simulink model "heaveCompMichael_v07"  (R2022b)
settings: Solver=VariableStepAuto  StartTime=0.0  StopTime=20  RelTol=1e-3
model workspace (MATLAB code in the model file):
  | %fluid data
  | rho = 875;
  | %valve config
  | P_r = 70e5;
  | Cd = 0.7;
  | Q_r = 200/6e4;
  | AdMax = Q_r/Cd/sqrt(2/rho*P_r/2);
  | 
  | g = 9.81;                   %gravity
  | zw = 0.8;                   %wave amplitude
  | tw = 10;                    %total wave period
  | ig = 46;                    %gear ratio gearbox
  | m = 9000;                   %mass of payload
  | mueq = 0.15;                %friction coeffisient
  | dd = 0.45;                  %diameter drum
  | nyv = 0.92;                 %volumetric effissiency
  | rd = dd/2;                  %radius drum
  | omega0 = 5;                 %velosity in friction equation
  | omegap = 1500;              %velosity hpu pump
  | nsh = 3;
  | gearrationsh = nsh.*2;
libraries: fl_lib x30, nesl_utility x18, sh_lib x4, slpidlib x1
settings Model: Creator=tolla  LastModifiedBy=marcu
settings SolverCC: MaxConsecutiveMinStep=10
settings DebuggingCC: UnconnectedInputMsg=warning  UnconnectedOutputMsg=warning  UnconnectedLineMsg=warning
settings ModelReferenceCC: EnableRefExpFcnMdlSchedulingChecks=on
settings RTWCC: DLArmComputeVersion=19.05

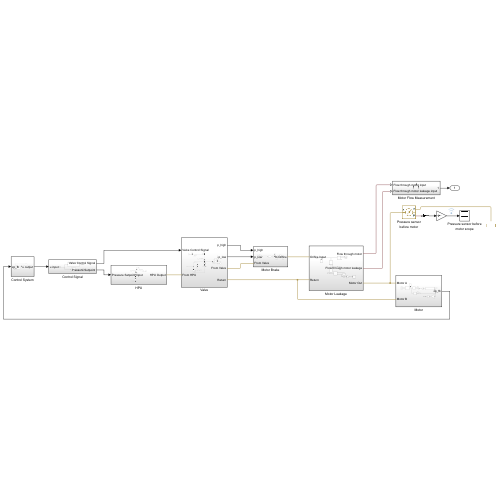
[thumbnail: Simulink's stored preview of the top-level diagram]
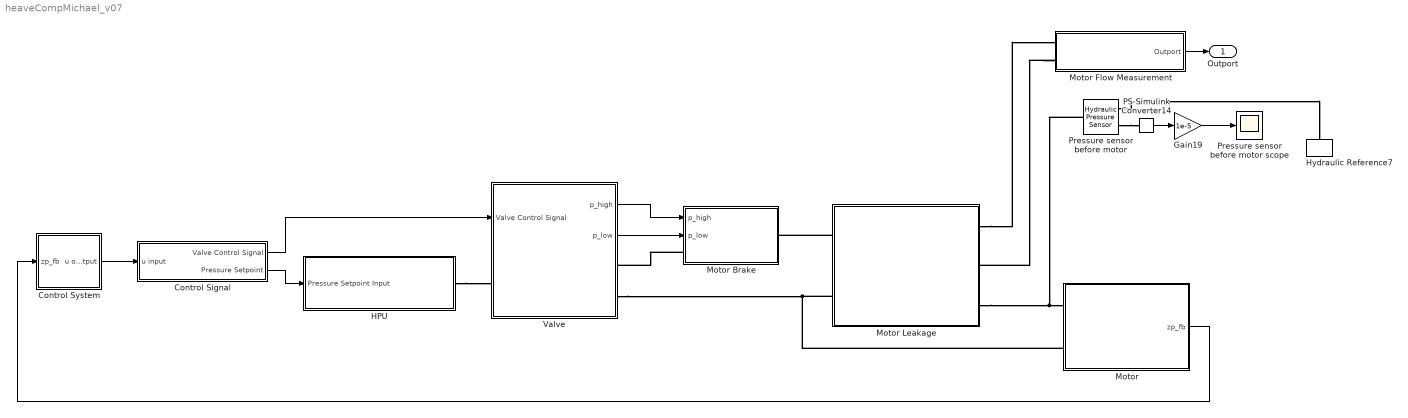
== system heaveCompMichael_v07 ==
  Control Signal : Subsystem
  Control System : Subsystem
  Gain19 : Gain  Gain=1e-5
  HPU : Subsystem
  Hydraulic Reference7 : fl_lib/Hydraulic/Hydraulic Elements/Hydraulic Reference
  Motor : Subsystem
  Motor Brake : Subsystem
  Motor Flow Measurement : Subsystem
  Motor Leakage : Subsystem
  PS-Simulink Converter14 : nesl_utility/PS-Simulink Converter  PhysicalDomain=network_engine_domain  SubClassName=ps_output  LeftPortType=input  RightPortType=output  PseudoPeriodic=off  Frequencies=[]  VectorFormat=inherit  Unit=inherit  AffineConversion=off
  Pressure sensor before motor : fl_lib/Hydraulic/Hydraulic Sensors/Hydraulic Pressure Sensor
  Pressure sensor before motor scope : Scope
  Valve : Subsystem
  Outport : Outport
  wires:
  PS-Simulink Converter14/1 -> Gain19/1
  Gain19/1 -> Pressure sensor before motor scope/1
  Motor/1(zp_fb) -> Control System/1(zp_fb)
  Valve/1(p_high) -> Motor Brake/1(p_high)
  Valve/2(p_low) -> Motor Brake/2(p_low)
  Motor Flow Measurement/1(Outport) -> Outport/1
  Control System/1(u output) -> Control Signal/1(u input)
  Control Signal/1(Valve Control Signal) -> Valve/1(Valve Control Signal)
  Control Signal/2(Pressure Setpoint) -> HPU/1(Pressure Setpoint Input)
  connections:
  Pressure sensor before motor/RConn1 -- Hydraulic Reference7/LConn1
  Pressure sensor before motor/RConn2 -- PS-Simulink Converter14/LConn1
  Motor/LConn2 -- Valve/RConn2 -- Motor Leakage/LConn2
  Motor Brake/LConn1 -- Valve/RConn1
  HPU/RConn1 -- Valve/LConn1
  Pressure sensor before motor/LConn1 -- Motor Leakage/RConn3 -- Motor/LConn1
  Motor Leakage/LConn1 -- Motor Brake/RConn1
  Motor Leakage/RConn1 -- Motor Flow Measurement/LConn1
  Motor Flow Measurement/LConn2 -- Motor Leakage/RConn2

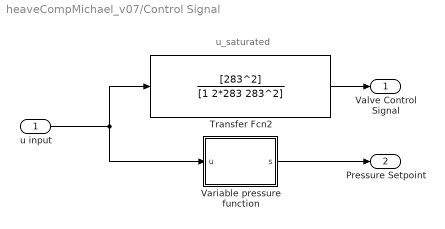
== system heaveCompMichael_v07/Control Signal ==
  note: u_saturated
  u input : Inport
  Transfer Fcn2 : TransferFcn  Numerator=[283^2]  Denominator=[1 2*283 283^2]
  Variable pressure function : MATLAB Function  TreatAsAtomicUnit=on
  Valve Control Signal : Outport
  Pressure Setpoint : Outport  Port=2
  wires:
  u input/1 -> Variable pressure function/1(u), Transfer Fcn2/1
  Variable pressure function/1(s) -> Pressure Setpoint/1
  Transfer Fcn2/1 -> Valve Control Signal/1

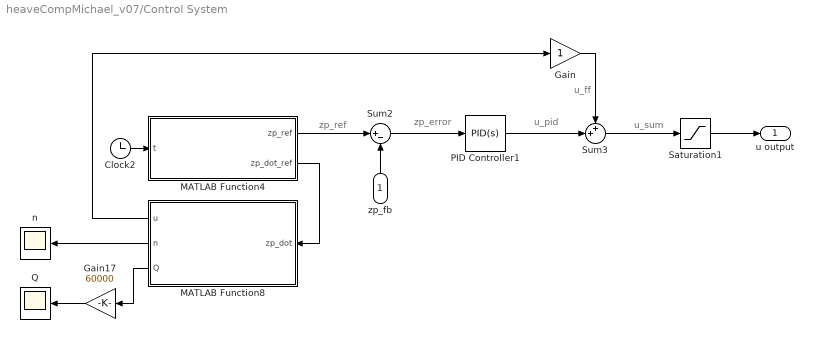
== system heaveCompMichael_v07/Control System ==
  note: u_ff
  note: u_sum
  note: u_pid
  note: zp_error
  note: zp_ref
  zp_fb : Inport
  Clock2 : Clock
  Gain : Gain
  Gain17 : Gain  Gain=60000
  MATLAB Function4 : MATLAB Function  TreatAsAtomicUnit=on
  MATLAB Function8 : MATLAB Function  TreatAsAtomicUnit=on
  PID Controller1 : slpidlib/PID Controller  Controller=PID  Form=Parallel  TimeDomain=Continuous-time  UseExternalTs=off  SampleTime=-1  IntegratorMethod=Forward Euler  FilterMethod=Forward Euler  ControllerParametersSource=internal  P=20  I=0  UseKiTs=off  D=0  N=100  UseFilter=on  TunerSelectOption=Transfer Function Based (PID Tuner App)  InitialConditionSource=internal  InitialConditionForIntegrator=0  InitialConditionForFilter=0  DifferentiatorICPrevScaledInput=0  ExternalReset=none  TrackingMode=off  Kt=1  LimitOutput=off  SatLimitsSource=internal  UpperSaturationLimit=inf  LowerSaturationLimit=-inf  LinearizeAsGain=on  AntiWindupMode=none  Kb=1  LimitIntegrator=off  UpperIntegratorSaturationLimit=inf  LowerIntegratorSaturationLimit=-inf  POutMin=[]  POutMax=[]  IOutMin=[]  IOutMax=[]  DOutMin=[]  DOutMax=[]  NOutMin=[]  NOutMax=[]  SumOutMin=[]  SumOutMax=[]  SaturationOutMin=[]  SaturationOutMax=[]  PParamMin=[]  PParamMax=[]  IParamMin=[]  IParamMax=[]  DParamMin=[]  DParamMax=[]  NParamMin=[]  NParamMax=[]  KbParamMin=[]  KbParamMax=[]  KtParamMin=[]  KtParamMax=[]  KbOutMin=[]  KbOutMax=[]  KtOutMin=[]  KtOutMax=[]  IntegratorOutMin=[]  IntegratorOutMax=[]  FilterOutMin=[]  FilterOutMax=[]  SumI1OutMin=[]  SumI1OutMax=[]  SumI2OutMin=[]  SumI2OutMax=[]  SumI3OutMin=[]  SumI3OutMax=[]  SumI4OutMin=[]  SumI4OutMax=[]  SumDOutMin=[]  SumDOutMax=[]  DifferentiatorOutMin=[]  DifferentiatorOutMax=[]  FilterDiffOutCoefMin=[]  FilterDiffOutCoefMax=[]  ReciprocalOutMin=[]  ReciprocalOutMax=[]  SumDenOutMin=[]  SumDenOutMax=[]  SumNumOutMin=[]  SumNumOutMax=[]  DivideOutMin=[]  DivideOutMax=[]  UdiffTsProdOutMin=[]  UdiffTsProdOutMax=[]  NTsProdOutMin=[]  NTsProdOutMax=[]  UintegralTsProdOutMin=[]  UintegralTsProdOutMax=[]  UngainTsProdOutMin=[]  UngainTsProdOutMax=[]  ClampingZeroOutDataTypeStr=Inherit: Inherit via back propagation  ClampingZeroOutMin=[]  ClampingZeroOutMax=[]  FilterDenConstantOutDataTypeStr=Inherit: Inherit via back propagation  FilterDenConstantOutMin=[]  FilterDenConstantOutMax=[]  PCopyOutDataTypeStr=Inherit: Inherit via back propagation  PCopyOutMin=[]  PCopyOutMax=[]  NCopyOutDataTypeStr=Inherit: Inherit via back propagation  NCopyOutMin=[]  NCopyOutMax=[]  IntegratorContinuousStateAttributes=''  IntegratorStateMustResolveToSignalObject=off  IntegratorRTWStateStorageClass=Auto  FilterContinuousStateAttributes=''  FilterStateMustResolveToSignalObject=off  FilterRTWStateStorageClass=Auto  ParallelPVariant=InternalParameters  IdealPVariant=Disabled  IVariant=InternalParameters  DVariant=InternalParameters  IntegratorVariant=Continuous  SatVariant=Disabled  AWVariant=Passthrough  PCopyVariant=Disabled  TRVariant=Disabled  FdbkBlocksVariant=Forward  IdealPFdbkVariant=Disabled  SatFdbkVariant=Disabled  DerivativeFilterVariant=ContFilter  NVariant=InternalParameters  NCopyVariant=Disabled  FilterICVariant=InternalICsFilter  IntegratorICVariant=InternalICs  ExternalResetVariant=Disabled  TRSumVariant=Passthrough  SumFdbkVariant=Disabled  SumVariant=Sum_PID  TsampFilterVariant=InternalTs  TsampNgainVariant=Passthrough  TsampIntegralVariant=Passthrough  ExternalSaturationOutDataTypeStr=Inherit: Same as second input
  Q : Scope
  Saturation1 : Saturate  UpperLimit=1  LowerLimit=-1
  Sum2 : Sum  Inputs=|+-
  Sum3 : Sum  Inputs=++|
  n : Scope
  u output : Outport
  wires:
  MATLAB Function8/3(Q) -> Gain17/1
  PID Controller1/1 -> Sum3/2
  MATLAB Function4/2(zp_dot_ref) -> MATLAB Function8/1(zp_dot)
  Gain17/1 -> Q/1
  Clock2/1 -> MATLAB Function4/1(t)
  MATLAB Function8/2(n) -> n/1
  Sum3/1 -> Saturation1/1
  zp_fb/1 -> Sum2/2
  MATLAB Function4/1(zp_ref) -> Sum2/1
  Sum2/1 -> PID Controller1/1
  MATLAB Function8/1(u) -> Gain/1
  Saturation1/1 -> u output/1
  Gain/1 -> Sum3/1

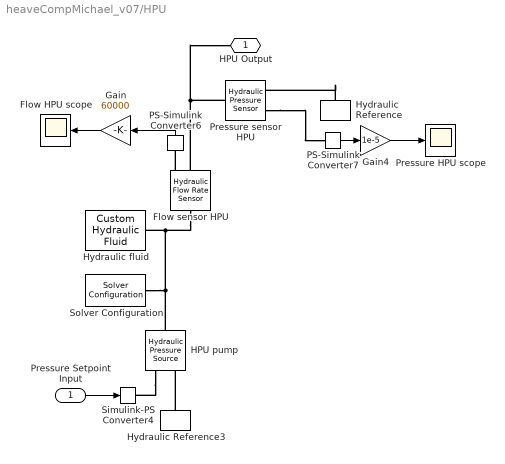
== system heaveCompMichael_v07/HPU ==
  Pressure Setpoint Input : Inport
  Flow HPU scope : Scope
  Flow sensor HPU : fl_lib/Hydraulic/Hydraulic Sensors/Hydraulic Flow Rate Sensor
  Gain : Gain  Gain=60000
  Gain4 : Gain  Gain=1e-5
  HPU pump : fl_lib/Hydraulic/Hydraulic Sources/Hydraulic Pressure Source
      settings: InternalSimscapePortConfiguration="{\"Bottom\":[],\"Left\":[{\"id\":\"P\",\"label\":\"P\",\"type\":\"foundation.hydraulic.hydraulic\"}],\"Right\":[{\"id\":\"S\",\"label\":\"S\",\"type\":\"input\"},{\"id\":\"T\",\"label\":\"T\",\"type\":\"foundation.hydraulic.hydraulic\"}],\"Top\":[]}"
  Hydraulic Reference : fl_lib/Hydraulic/Hydraulic Elements/Hydraulic Reference
  Hydraulic Reference3 : fl_lib/Hydraulic/Hydraulic Elements/Hydraulic Reference
  Hydraulic fluid : fl_lib/Hydraulic/Hydraulic Utilities/Custom Hydraulic Fluid  density=875 kg/m^3  viscosity_kin=18e-6 m^2/s  bulk=1100 MPa  alpha=0.005  range_error=2
      settings: InternalSimscapePortConfiguration="{\"Bottom\":[],\"Left\":[],\"Right\":[{\"id\":\"G\",\"label\":\"\",\"type\":\"foundation.hydraulic.hydraulic\"}],\"Top\":[]}"
  PS-Simulink Converter6 : nesl_utility/PS-Simulink Converter  PhysicalDomain=network_engine_domain  SubClassName=ps_output  LeftPortType=input  RightPortType=output  PseudoPeriodic=off  Frequencies=[]  VectorFormat=inherit  Unit=inherit  AffineConversion=off
  PS-Simulink Converter7 : nesl_utility/PS-Simulink Converter  PhysicalDomain=network_engine_domain  SubClassName=ps_output  LeftPortType=input  RightPortType=output  PseudoPeriodic=off  Frequencies=[]  VectorFormat=inherit  Unit=inherit  AffineConversion=off
  Pressure HPU scope : Scope
  Pressure sensor HPU : fl_lib/Hydraulic/Hydraulic Sensors/Hydraulic Pressure Sensor
  Simulink-PS Converter4 : nesl_utility/Simulink-PS Converter  PhysicalDomain=network_engine_domain  SubClassName=ps_input  LeftPortType=input  RightPortType=output  PseudoPeriodic=off  Frequencies=[]  NoiseDistribution=none  NoiseParameters=[]  Unit=1  AffineConversion=off  FilteringAndDerivatives=provide  SimscapeFilterOrder=1  InputFilterTimeConstant=0.001  UdotUserProvided=0
  Solver Configuration : nesl_utility/Solver Configuration  PhysicalDomain=network_engine_domain  SubClassName=solver  LeftPortType=input  RightPortType=generic  Tones=[]  Harmonics=[]  SimulateNoise=off  Profile=off  UseLocalSampling=off  EnableSwitchedLinearOptims=on  FrequencyDomain=off  UseCCode=off  RelTol=0.001  AbsTol=1e-06  MinStep=1e-09  ToWorkspace=off  RevertToSquareIcSolve=off  NumHomotopyIterations=100  PhasorMode=off  PhasorModeNumHarmonics=1  ConsistencySolver=NEWTON_FTOL  IndexReductionMethod=DerivativeReplacement  DoDC=off  ResidualTolerance=1e-09  ConsistencyTolSource=GLOBAL  ConsistencyAbsTol=0.001  ConsistencyRelTol=0.001  ConsistencyTolFactor=0.001  UseLocalSolver=off  LocalSolverChoice=NE_BACKWARD_EULER_ADVANCER  ResolveIndetEquations=on  FunctionEvalNumThread=1  LocalSolverSampleTime=0.001  DoFixedCost=off  MaxNonlinIter=3  MaxModeIter=2  ComputeImpulses=off  ImpulseIterations=2  LinearAlgebra=auto  LinearAlgebraNumThread=0  EquationFormulation=NE_TIME_EF  DelaysMemoryBudget=1024  AutomaticFiltering=on  FilteringTimeConstant=0.001  PartitionStorageMethod=AS_NEEDED  PartitionMemoryBudget=1024  PartitionMethod=ROBUST
  HPU Output : PMIOPort  Side=Right
  wires:
  PS-Simulink Converter6/1 -> Gain/1
  PS-Simulink Converter7/1 -> Gain4/1
  Pressure Setpoint Input/1 -> Simulink-PS Converter4/1
  Gain/1 -> Flow HPU scope/1
  Gain4/1 -> Pressure HPU scope/1
  connections:
  HPU pump/LConn1 -- Solver Configuration/RConn1 -- Hydraulic fluid/RConn1 -- Flow sensor HPU/LConn1
  Hydraulic Reference3/LConn1 -- HPU pump/RConn2
  HPU pump/RConn1 -- Simulink-PS Converter4/RConn1
  Pressure sensor HPU/RConn2 -- PS-Simulink Converter7/LConn1
  Flow sensor HPU/RConn1 -- PS-Simulink Converter6/LConn1
  Flow sensor HPU/RConn2 -- Pressure sensor HPU/LConn1 -- HPU Output/RConn1
  Hydraulic Reference/LConn1 -- Pressure sensor HPU/RConn1

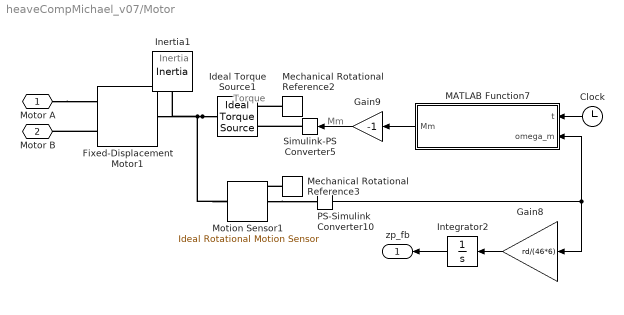
== system heaveCompMichael_v07/Motor ==
  note: Torque
  note: Inertia
  note: Mm
  Clock : Clock
  Fixed-Displacement Motor1 : sh_lib/Pumps and Motors/Fixed-Displacement Motor  D=28.1 cm^3/rev  loss_spec=1  w_nominal=616 rad/s  pr_nominal=185 bar  visc_nominal=18 cSt  dens_nominal=875 kg/m^3  efficiency_vol=1  no_load_torque=0 N*m  torque_pressure_coeff=0 N*m/Pa  p_diff_eff_TLU=[100000, 1000000, 2000000] Pa  omega_eff_TLU=[25, 50, 100, 200, 300, 400] rad/s  vol_eff_TLU=[.816, .908, .954, .977, .981, .984; .325, .663, .831, .916, .925, .946; .137, .568, .78, .892, .893, .91]  mech_eff_TLU=[.996, .996, .996, .996, .996, .996; .988, .989, .989, .989, .989, .99; .981, .981, .982, .982, .983, .984]  p_diff_loss_TLU=[100000, 1000000, 2000000] Pa  omega_loss_TLU=[25, 50, 100, 200, 300, 400] rad/s  vol_loss_TLU=[.0282, .0253, .0241, .0235, .0291, .0325; .2596, .1271, .1017, .0917, .1216, .1142; .7874, .1901, .141, .1211, .1797, .1978] * 1e-3 m^3/s  mech_loss_TLU=[.002, .002, .002, .002, .002, .002; .06, .055, .055, .055, .055, .05; .19, .19, .18, .18, .17, .16] N*m  pressure_threshold=1e5 Pa  omega_threshold=10 rad/s  quadrant_check=0  pressure_check=0  min_valid_pressure=0 Pa  vol_eff_min=1e-3  vol_eff_max=1  mech_eff_min=1e-3  mech_eff_max=1
      settings: InternalSimscapePortConfiguration="{\"Bottom\":[],\"Left\":[{\"id\":\"A\",\"label\":\"A\",\"type\":\"foundation.hydraulic.hydraulic\"},{\"id\":\"B\",\"label\":\"B\",\"type\":\"foundation.hydraulic.hydraulic\"}],\"Right\":[{\"id\":\"S\",\"label\":\"S\",\"type\":\"foundation.mechanical.rotational.rotational\"}],\"Top\":[]}"
  Gain8 : Gain  Gain=rd/(46*6)
  Gain9 : Gain  Gain=-1
  Ideal Torque Source1 : fl_lib/Mechanical/Mechanical Sources/Ideal Torque Source
  Inertia1 : fl_lib/Mechanical/Rotational Elements/Inertia  Tag=Factory Generic  inertia=0.0072 kg*m^2  num_ports=foundation.enum.numPorts2.one  w_specify=off  w_priority=High  w=0 rad/s  w_nominal_specify=off  w_nominal_unit=rad/s  w_nominal_value=1  t_specify=off  t_priority=High  t=0 N*m  t_nominal_specify=off  t_nominal_unit=N*m  t_nominal_value=1
  Integrator2 : Integrator
  MATLAB Function7 : MATLAB Function  TreatAsAtomicUnit=on
  Mechanical Rotational Reference2 : fl_lib/Mechanical/Rotational Elements/Mechanical Rotational Reference
  Mechanical Rotational Reference3 : fl_lib/Mechanical/Rotational Elements/Mechanical Rotational Reference
  Motion Sensor1 : fl_lib/Mechanical/Mechanical Sensors/Ideal Rotational Motion Sensor  Tag=Factory Generic  reference=foundation.enum.MeasurementReference.difference  acceleration_port=false  velocity_port=true  position_port=true  wrap_angle=simscape.enum.onoff.on  offset=0 rad
  PS-Simulink Converter10 : nesl_utility/PS-Simulink Converter  PhysicalDomain=network_engine_domain  SubClassName=ps_output  LeftPortType=input  RightPortType=output  PseudoPeriodic=off  Frequencies=[]  VectorFormat=inherit  Unit=inherit  AffineConversion=off
  Simulink-PS Converter5 : nesl_utility/Simulink-PS Converter  PhysicalDomain=network_engine_domain  SubClassName=ps_input  LeftPortType=input  RightPortType=output  PseudoPeriodic=off  Frequencies=[]  NoiseDistribution=none  NoiseParameters=[]  Unit=1  AffineConversion=off  FilteringAndDerivatives=provide  SimscapeFilterOrder=1  InputFilterTimeConstant=0.001  UdotUserProvided=0
  Motor A : PMIOPort  Side=Left
  Motor B : PMIOPort  Port=2  Side=Left
  zp_fb : Outport
  wires:
  MATLAB Function7/1(Mm) -> Gain9/1
  Gain8/1 -> Integrator2/1
  Integrator2/1 -> zp_fb/1
  PS-Simulink Converter10/1 -> MATLAB Function7/2(omega_m), Gain8/1
  Gain9/1 -> Simulink-PS Converter5/1
  Clock/1 -> MATLAB Function7/1(t)
  connections:
  Simulink-PS Converter5/RConn1 -- Ideal Torque Source1/RConn1
  Ideal Torque Source1/LConn1 -- Fixed-Displacement Motor1/RConn1 -- Inertia1/LConn1 -- Motion Sensor1/LConn1
  Motor A/RConn1 -- Fixed-Displacement Motor1/LConn1
  Mechanical Rotational Reference2/LConn1 -- Ideal Torque Source1/RConn2
  Mechanical Rotational Reference3/LConn1 -- Motion Sensor1/RConn1
  Motion Sensor1/RConn2 -- PS-Simulink Converter10/LConn1
  Fixed-Displacement Motor1/LConn2 -- Motor B/RConn1

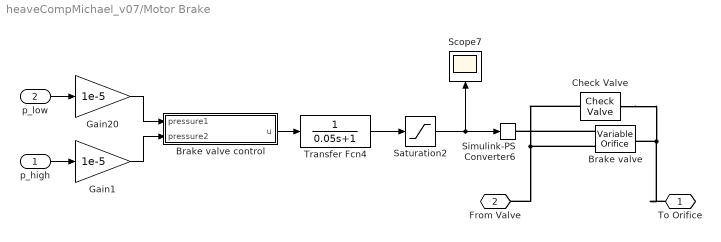
== system heaveCompMichael_v07/Motor Brake ==
  p_high : Inport
  p_low : Inport  Port=2
  Brake valve : sh_lib/Orifices/Variable Orifice  mdl_type=1  area_max=1.7928e-4 m^2  opening_max=1 m  opening_tab=[-.002, 0, .002, .005, .015] m  area_tab=[1e-09, 2.0352e-07, 4.0736e-05, .00011438, .00034356] m^2  pressure_tab=[-10000000, -5000000, -2000000, 2000000, 5000000, 10000000] Pa  flow_rate_tab=[-1e-07, -7.0711e-08, -4.4721e-08, 4.4721e-08, 7.0711e-08, 1e-07; -2.0352e-05, -1.4391e-05, -9.1017e-06, 9.1017e-06, 1.4391e-05, 2.0352e-05; -.0040736, -.0028805, -.0018218, .0018218, .0028805, .0040736; -.011438, -.0080879, -.0051152, .0051152, .0080879, .011438; -.034356, -.024293, -.015364, .015364, .024293, .034356] m^3/s  interp_method=1  extrap_method=1  or=1  C_d=0.7  x_0=0 m  A_leak=1e-13 m^2  lam_spec=1  B_lam=0.999  Re_cr=12  flow_rate_specify=off  flow_rate_priority=None  flow_rate=0 m^3/s  flow_rate_nominal_specify=off  flow_rate_nominal_unit=m^3/s  flow_rate_nominal_value=1  pressure_drop_specify=off  pressure_drop_priority=None  pressure_drop=0 Pa  pressure_drop_nominal_specify=off  pressure_drop_nominal_unit=Pa  pressure_drop_nominal_value=1
      settings: InternalSimscapePortConfiguration="{\"Bottom\":[],\"Left\":[{\"id\":\"S\",\"label\":\"S\",\"type\":\"input\"},{\"id\":\"A\",\"label\":\"A\",\"type\":\"foundation.hydraulic.hydraulic\"}],\"Right\":[{\"id\":\"B\",\"label\":\"B\",\"type\":\"foundation.hydraulic.hydraulic\"}],\"Top\":[]}"
  Brake valve control : MATLAB Function  TreatAsAtomicUnit=on
  Check Valve : sh_lib/Valves/Directional Valves/Check Valve  area_max=200 mm^2  pres_crack=0.3e5 Pa  pres_max=1.2e5 Pa  C_d=0.7  A_leak=1e-12 m^2  lam_spec=1  B_lam=0.999  Re_cr=12  dynamic=0  tau=0.1 s  area_init=1e-12 m^2
      settings: InternalSimscapePortConfiguration="{\"Bottom\":[],\"Left\":[{\"id\":\"A\",\"label\":\"A\",\"type\":\"foundation.hydraulic.hydraulic\"}],\"Right\":[{\"id\":\"B\",\"label\":\"B\",\"type\":\"foundation.hydraulic.hydraulic\"}],\"Top\":[]}"
  Gain1 : Gain  Gain=1e-5
  Gain20 : Gain  Gain=1e-5
  Saturation2 : Saturate  UpperLimit=1  LowerLimit=0
  Scope7 : Scope
  Simulink-PS Converter6 : nesl_utility/Simulink-PS Converter  PhysicalDomain=network_engine_domain  SubClassName=ps_input  LeftPortType=input  RightPortType=output  PseudoPeriodic=off  Frequencies=[]  NoiseDistribution=none  NoiseParameters=[]  Unit=1  AffineConversion=off  FilteringAndDerivatives=provide  SimscapeFilterOrder=1  InputFilterTimeConstant=0.001  UdotUserProvided=0
  Transfer Fcn4 : TransferFcn  Denominator=[0.05 1]
  To Orifice : PMIOPort  Side=Right
  From Valve : PMIOPort  Port=2  Side=Left
  wires:
  p_low/1 -> Gain20/1
  Brake valve control/1(u) -> Transfer Fcn4/1
  Saturation2/1 -> Scope7/1, Simulink-PS Converter6/1
  Gain20/1 -> Brake valve control/1(pressure1)
  Transfer Fcn4/1 -> Saturation2/1
  p_high/1 -> Gain1/1
  Gain1/1 -> Brake valve control/2(pressure2)
  connections:
  Check Valve/RConn1 -- To Orifice/RConn1 -- Brake valve/RConn1
  Brake valve/LConn2 -- Check Valve/LConn1 -- From Valve/RConn1
  Brake valve/LConn1 -- Simulink-PS Converter6/RConn1

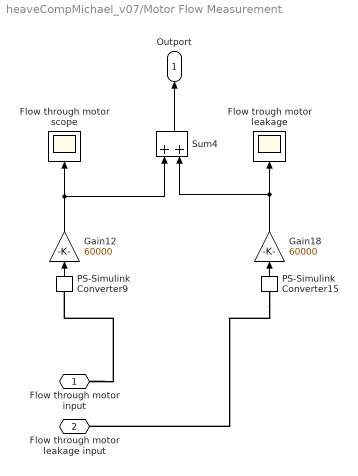
== system heaveCompMichael_v07/Motor Flow Measurement ==
  Flow through motor scope : Scope
  Flow trough motor leakage : Scope
  Gain12 : Gain  Gain=60000
  Gain18 : Gain  Gain=60000
  PS-Simulink Converter15 : nesl_utility/PS-Simulink Converter  PhysicalDomain=network_engine_domain  SubClassName=ps_output  LeftPortType=input  RightPortType=output  PseudoPeriodic=off  Frequencies=[]  VectorFormat=inherit  Unit=inherit  AffineConversion=off
  PS-Simulink Converter9 : nesl_utility/PS-Simulink Converter  PhysicalDomain=network_engine_domain  SubClassName=ps_output  LeftPortType=input  RightPortType=output  PseudoPeriodic=off  Frequencies=[]  VectorFormat=inherit  Unit=inherit  AffineConversion=off
  Sum4 : Sum
  Flow through motor input : PMIOPort  Side=Left
  Flow through motor leakage input : PMIOPort  Port=2  Side=Left
  Outport : Outport
  wires:
  Gain18/1 -> Sum4/2, Flow trough motor leakage/1
  PS-Simulink Converter9/1 -> Gain12/1
  Gain12/1 -> Flow through motor scope/1, Sum4/1
  PS-Simulink Converter15/1 -> Gain18/1
  Sum4/1 -> Outport/1
  connections:
  PS-Simulink Converter15/LConn1 -- Flow through motor leakage input/RConn1
  Flow through motor input/RConn1 -- PS-Simulink Converter9/LConn1

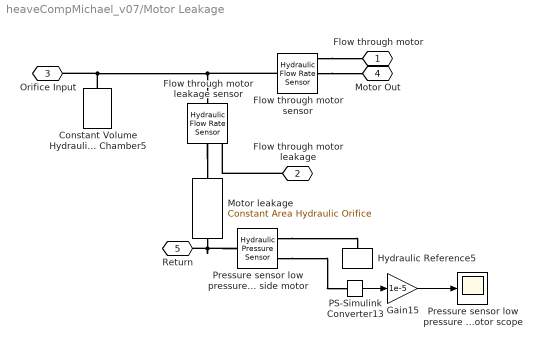
== system heaveCompMichael_v07/Motor Leakage ==
  Constant Volume Hydraulic Chamber5 : fl_lib/Hydraulic/Hydraulic Elements/Constant Volume Hydraulic Chamber  ch_sp=foundation.enum.chamberGeometry.volume  wall_type=foundation.enum.chamber_spec.rigid  ch_volume=10 cm^3  d_in=1e-2 m  length=1 m  pr_r_coef=1.2e-12 m/Pa  time_const=0.01 s  k_sh=1.4  pressure_specify=on  pressure_priority=High  pressure=150 bar  pressure_nominal_specify=off  pressure_nominal_unit=Pa  pressure_nominal_value=1  diameter_incr_specify=off  diameter_incr_priority=High  diameter_incr=0 m  diameter_incr_nominal_specify=off  diameter_incr_nominal_unit=m  diameter_incr_nominal_value=1  flow_rate_specify=off  flow_rate_priority=None  flow_rate=1e-3 m^3/s  flow_rate_nominal_specify=off  flow_rate_nominal_unit=m^3/s  flow_rate_nominal_value=1
      settings: InternalSimscapePortConfiguration="{\"Bottom\":[],\"Left\":[{\"id\":\"A\",\"label\":\"\",\"type\":\"foundation.hydraulic.hydraulic\"}],\"Right\":[],\"Top\":[]}"
  Flow through motor leakage sensor : fl_lib/Hydraulic/Hydraulic Sensors/Hydraulic Flow Rate Sensor
  Flow through motor sensor : fl_lib/Hydraulic/Hydraulic Sensors/Hydraulic Flow Rate Sensor
  Gain15 : Gain  Gain=1e-5
  Hydraulic Reference5 : fl_lib/Hydraulic/Hydraulic Elements/Hydraulic Reference
  Motor leakage : fl_lib/Hydraulic/Hydraulic Elements/Constant Area Hydraulic Orifice  area=1.12 mm^2  C_d=0.7  lam_spec=1  B_lam=0.999  Re_cr=12  q_specify=off  q_priority=None  q=1e-3 m^3/s  q_nominal_specify=off  q_nominal_unit=m^3/s  q_nominal_value=1  p_specify=off  p_priority=None  p=0 Pa  p_nominal_specify=off  p_nominal_unit=Pa  p_nominal_value=1
      settings: InternalSimscapePortConfiguration="{\"Bottom\":[],\"Left\":[{\"id\":\"A\",\"label\":\"A\",\"type\":\"foundation.hydraulic.hydraulic\"}],\"Right\":[{\"id\":\"B\",\"label\":\"B\",\"type\":\"foundation.hydraulic.hydraulic\"}],\"Top\":[]}"
  PS-Simulink Converter13 : nesl_utility/PS-Simulink Converter  PhysicalDomain=network_engine_domain  SubClassName=ps_output  LeftPortType=input  RightPortType=output  PseudoPeriodic=off  Frequencies=[]  VectorFormat=inherit  Unit=inherit  AffineConversion=off
  Pressure sensor low pressure side motor : fl_lib/Hydraulic/Hydraulic Sensors/Hydraulic Pressure Sensor
  Pressure sensor low pressure side motor scope : Scope
  Flow through motor : PMIOPort  Side=Right
  Flow through motor leakage : PMIOPort  Port=2  Side=Right
  Orifice Input : PMIOPort  Port=3  Side=Left
  Motor Out : PMIOPort  Port=4  Side=Right
  Return : PMIOPort  Port=5  Side=Left
  wires:
  PS-Simulink Converter13/1 -> Gain15/1
  Gain15/1 -> Pressure sensor low pressure side motor scope/1
  connections:
  Flow through motor leakage/RConn1 -- Flow through motor leakage sensor/RConn1
  Flow through motor leakage sensor/RConn2 -- Motor leakage/LConn1
  Constant Volume Hydraulic Chamber5/LConn1 -- Orifice Input/RConn1 -- Flow through motor leakage sensor/LConn1 -- Flow through motor sensor/LConn1
  Flow through motor sensor/RConn1 -- Flow through motor/RConn1
  Pressure sensor low pressure side motor/RConn1 -- Hydraulic Reference5/LConn1
  Pressure sensor low pressure side motor/RConn2 -- PS-Simulink Converter13/LConn1
  Flow through motor sensor/RConn2 -- Motor Out/RConn1
  Pressure sensor low pressure side motor/LConn1 -- Motor leakage/RConn1 -- Return/RConn1

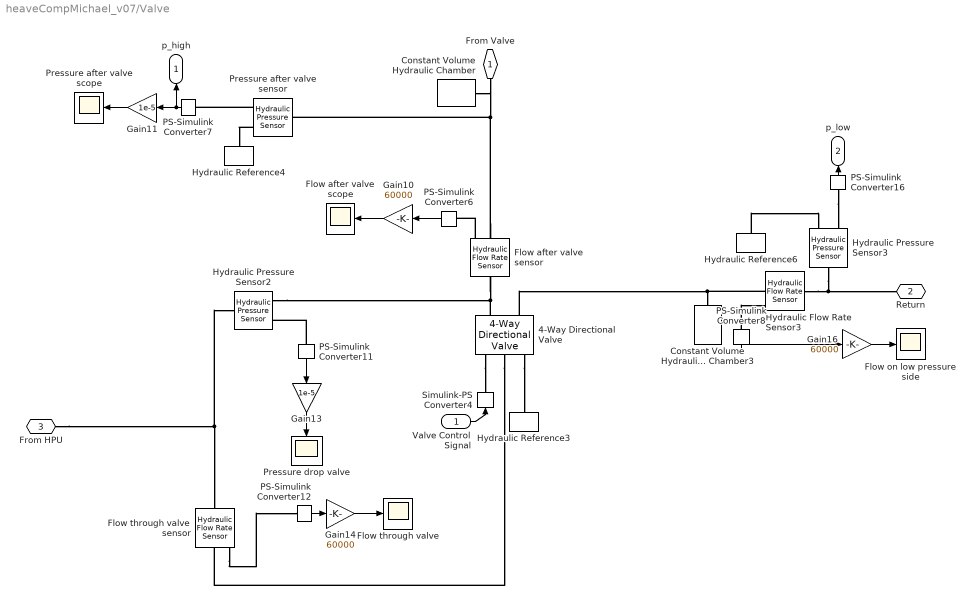
== system heaveCompMichael_v07/Valve ==
  Valve Control Signal : Inport
  4-Way Directional Valve : sh_lib/Valves/Directional Valves/4-Way Directional Valve  area_spec=sh.valves.directional_valves.enum.area_spec.identical  mdl_type_identical=sh.valves.directional_valves.enum.mdl_type.linear  mdl_type_different=sh.valves.directional_valves.enum.mdl_type.linear  interp_method_identical=sh.valves.directional_valves.enum.interp_method.linear  interp_method_different=sh.valves.directional_valves.enum.interp_method.linear  extrap_method_identical=sh.valves.directional_valves.enum.extrap_method.linear  extrap_method_different=sh.valves.directional_valves.enum.extrap_method.linear  A_leak=1e-12 m^2  C_d=0.7  lam_spec=sh.valves.directional_valves.enum.lam_spec.pressure_ratio  B_lam=0.999  Re_cr=12  opening_max=1 m  area_max=5.324e-5 m^2  opening_max_P_A=0.005 m  area_max_P_A=0.5e-4 m^2  opening_max_P_B=0.005 m  area_max_P_B=0.5e-4 m^2  opening_max_A_T=0.005 m  area_max_A_T=0.5e-4 m^2  opening_max_B_T=0.005 m  area_max_B_T=0.5e-4 m^2  opening_area_tab=[-.002, 0, .002, .005, .015] m  area_tab=[1e-09, 2.0352e-07, 4.0736e-05, .00011438, .00034356] m^2  opening_flow_rate_tab=[-.002, 0, .002, .005, .015] m  pressure_tab=[-10000000, -5000000, -2000000, 2000000, 5000000, 10000000] Pa  flow_rate_tab=[-1e-07, -7.0711e-08, -4.4721e-08, 4.4721e-08, 7.0711e-08, 1e-07; -2.0352e-05, -1.4391e-05, -9.1017e-06, 9.1017e-06, 1.4391e-05, 2.0352e-05; -.0040736, -.0028805, -.0018218, .0018218, .0028805, .0040736; -.011438, -.0080879, -.0051152, .0051152, .0080879, .011438; -.034356, -.024293, -.015364, .015364, .024293, .034356] m^3/s  opening_area_tab_P_A=[-.002, 0, .002, .005, .015] m  area_tab_P_A=[1e-09, 2.0352e-07, 4.0736e-05, .00011438, .00034356] m^2  opening_flow_rate_tab_P_A=[-.002, 0, .002, .005, .015] m  pressure_tab_P_A=[-10000000, -5000000, -2000000, 2000000, 5000000, 10000000] Pa  flow_rate_tab_P_A=[-1e-07, -7.0711e-08, -4.4721e-08, 4.4721e-08, 7.0711e-08, 1e-07; -2.0352e-05, -1.4391e-05, -9.1017e-06, 9.1017e-06, 1.4391e-05, 2.0352e-05; -.0040736, -.0028805, -.0018218, .0018218, .0028805, .0040736; -.011438, -.0080879, -.0051152, .0051152, .0080879, .011438; -.034356, -.024293, -.015364, .015364, .024293, .034356] m^3/s  opening_area_tab_P_B=[-.002, 0, .002, .005, .015] m  area_tab_P_B=[1e-09, 2.0352e-07, 4.0736e-05, .00011438, .00034356] m^2  opening_flow_rate_tab_P_B=[-.002, 0, .002, .005, .015] m  pressure_tab_P_B=[-10000000, -5000000, -2000000, 2000000, 5000000, 10000000] Pa  flow_rate_tab_P_B=[-1e-07, -7.0711e-08, -4.4721e-08, 4.4721e-08, 7.0711e-08, 1e-07; -2.0352e-05, -1.4391e-05, -9.1017e-06, 9.1017e-06, 1.4391e-05, 2.0352e-05; -.0040736, -.0028805, -.0018218, .0018218, .0028805, .0040736; -.011438, -.0080879, -.0051152, .0051152, .0080879, .011438; -.034356, -.024293, -.015364, .015364, .024293, .034356] m^3/s  opening_area_tab_A_T=[-.002, 0, .002, .005, .015] m  area_tab_A_T=[1e-09, 2.0352e-07, 4.0736e-05, .00011438, .00034356] m^2  opening_flow_rate_tab_A_T=[-.002, 0, .002, .005, .015] m  pressure_tab_A_T=[-10000000, -5000000, -2000000, 2000000, 5000000, 10000000] Pa  flow_rate_tab_A_T=[-1e-07, -7.0711e-08, -4.4721e-08, 4.4721e-08, 7.0711e-08, 1e-07; -2.0352e-05, -1.4391e-05, -9.1017e-06, 9.1017e-06, 1.4391e-05, 2.0352e-05; -.0040736, -.0028805, -.0018218, .0018218, .0028805, .0040736; -.011438, -.0080879, -.0051152, .0051152, .0080879, .011438; -.034356, -.024293, -.015364, .015364, .024293, .034356] m^3/s  opening_area_tab_B_T=[-.002, 0, .002, .005, .015] m  area_tab_B_T=[1e-09, 2.0352e-07, 4.0736e-05, .00011438, .00034356] m^2  opening_flow_rate_tab_B_T=[-.002, 0, .002, .005, .015] m  pressure_tab_B_T=[-10000000, -5000000, -2000000, 2000000, 5000000, 10000000] Pa  flow_rate_tab_B_T=[-1e-07, -7.0711e-08, -4.4721e-08, 4.4721e-08, 7.0711e-08, 1e-07; -2.0352e-05, -1.4391e-05, -9.1017e-06, 9.1017e-06, 1.4391e-05, 2.0352e-05; -.0040736, -.0028805, -.0018218, .0018218, .0028805, .0040736; -.011438, -.0080879, -.0051152, .0051152, .0080879, .011438; -.034356, -.024293, -.015364, .015364, .024293, .034356] m^3/s  x_0_P_A=0 m  x_0_P_B=0 m  x_0_A_T=0 m  x_0_B_T=0 m
      settings: InternalSimscapePortConfiguration="{\"Bottom\":[],\"Left\":[{\"id\":\"A\",\"label\":\"A\",\"type\":\"foundation.hydraulic.hydraulic\"},{\"id\":\"B\",\"label\":\"B\",\"type\":\"foundation.hydraulic.hydraulic\"}],\"Right\":[{\"id\":\"S\",\"label\":\"S\",\"type\":\"input\"},{\"id\":\"P\",\"label\":\"P\",\"type\":\"foundation.hydraulic.hydraulic\"},{\"id\":\"T\",\"label\":\"T\",\"type\":\"foundation.hydraulic.hydraulic\"}],\"Top\":[]}"
  Constant Volume Hydraulic Chamber : fl_lib/Hydraulic/Hydraulic Elements/Constant Volume Hydraulic Chamber  ch_sp=foundation.enum.chamberGeometry.volume  wall_type=foundation.enum.chamber_spec.rigid  ch_volume=10 cm^3  d_in=1e-2 m  length=1 m  pr_r_coef=1.2e-12 m/Pa  time_const=0.01 s  k_sh=1.4  pressure_specify=on  pressure_priority=High  pressure=150 bar  pressure_nominal_specify=off  pressure_nominal_unit=Pa  pressure_nominal_value=1  diameter_incr_specify=off  diameter_incr_priority=High  diameter_incr=0 m  diameter_incr_nominal_specify=off  diameter_incr_nominal_unit=m  diameter_incr_nominal_value=1  flow_rate_specify=off  flow_rate_priority=None  flow_rate=1e-3 m^3/s  flow_rate_nominal_specify=off  flow_rate_nominal_unit=m^3/s  flow_rate_nominal_value=1
      settings: InternalSimscapePortConfiguration="{\"Bottom\":[],\"Left\":[{\"id\":\"A\",\"label\":\"\",\"type\":\"foundation.hydraulic.hydraulic\"}],\"Right\":[],\"Top\":[]}"
  Constant Volume Hydraulic Chamber3 : fl_lib/Hydraulic/Hydraulic Elements/Constant Volume Hydraulic Chamber  ch_sp=foundation.enum.chamberGeometry.volume  wall_type=foundation.enum.chamber_spec.rigid  ch_volume=10 cm^3  d_in=1e-2 m  length=1 m  pr_r_coef=1.2e-12 m/Pa  time_const=0.01 s  k_sh=1.4  pressure_specify=on  pressure_priority=High  pressure=20 bar  pressure_nominal_specify=off  pressure_nominal_unit=Pa  pressure_nominal_value=1  diameter_incr_specify=off  diameter_incr_priority=High  diameter_incr=0 m  diameter_incr_nominal_specify=off  diameter_incr_nominal_unit=m  diameter_incr_nominal_value=1  flow_rate_specify=off  flow_rate_priority=None  flow_rate=1e-3 m^3/s  flow_rate_nominal_specify=off  flow_rate_nominal_unit=m^3/s  flow_rate_nominal_value=1
      settings: InternalSimscapePortConfiguration="{\"Bottom\":[],\"Left\":[{\"id\":\"A\",\"label\":\"\",\"type\":\"foundation.hydraulic.hydraulic\"}],\"Right\":[],\"Top\":[]}"
  Flow after valve scope : Scope
  Flow after valve sensor : fl_lib/Hydraulic/Hydraulic Sensors/Hydraulic Flow Rate Sensor
  Flow on low pressure side : Scope
  Flow through valve : Scope
  Flow through valve sensor : fl_lib/Hydraulic/Hydraulic Sensors/Hydraulic Flow Rate Sensor
  Gain10 : Gain  Gain=60000
  Gain11 : Gain  Gain=1e-5
  Gain13 : Gain  Gain=1e-5
  Gain14 : Gain  Gain=60000
  Gain16 : Gain  Gain=60000
  Hydraulic Flow Rate Sensor3 : fl_lib/Hydraulic/Hydraulic Sensors/Hydraulic Flow Rate Sensor
  Hydraulic Pressure Sensor2 : fl_lib/Hydraulic/Hydraulic Sensors/Hydraulic Pressure Sensor
  Hydraulic Pressure Sensor3 : fl_lib/Hydraulic/Hydraulic Sensors/Hydraulic Pressure Sensor
  Hydraulic Reference3 : fl_lib/Hydraulic/Hydraulic Elements/Hydraulic Reference
  Hydraulic Reference4 : fl_lib/Hydraulic/Hydraulic Elements/Hydraulic Reference
  Hydraulic Reference6 : fl_lib/Hydraulic/Hydraulic Elements/Hydraulic Reference
  PS-Simulink Converter{6..8,11..12,16} (6 alike) : nesl_utility/PS-Simulink Converter  PhysicalDomain=network_engine_domain  SubClassName=ps_output  LeftPortType=input  RightPortType=output  PseudoPeriodic=off  Frequencies=[]  VectorFormat=inherit  Unit=inherit  AffineConversion=off
  Pressure drop valve : Scope
  Pressure after valve scope : Scope
  Pressure after valve sensor : fl_lib/Hydraulic/Hydraulic Sensors/Hydraulic Pressure Sensor
  Simulink-PS Converter4 : nesl_utility/Simulink-PS Converter  PhysicalDomain=network_engine_domain  SubClassName=ps_input  LeftPortType=input  RightPortType=output  PseudoPeriodic=off  Frequencies=[]  NoiseDistribution=none  NoiseParameters=[]  Unit=1  AffineConversion=off  FilteringAndDerivatives=provide  SimscapeFilterOrder=1  InputFilterTimeConstant=0.001  UdotUserProvided=0
  From Valve : PMIOPort  Side=Right
  Return : PMIOPort  Port=2  Side=Right
  From HPU : PMIOPort  Port=3  Side=Left
  p_high : Outport
  p_low : Outport  Port=2
  wires:
  PS-Simulink Converter16/1 -> p_low/1
  Gain16/1 -> Flow on low pressure side/1
  PS-Simulink Converter7/1 -> p_high/1, Gain11/1
  PS-Simulink Converter8/1 -> Gain16/1
  Gain11/1 -> Pressure after valve scope/1
  PS-Simulink Converter6/1 -> Gain10/1
  Gain10/1 -> Flow after valve scope/1
  PS-Simulink Converter12/1 -> Gain14/1
  Gain13/1 -> Pressure drop valve/1
  PS-Simulink Converter11/1 -> Gain13/1
  Gain14/1 -> Flow through valve/1
  Valve Control Signal/1 -> Simulink-PS Converter4/1
  connections:
  Hydraulic Flow Rate Sensor3/LConn1 -- Hydraulic Pressure Sensor3/LConn1 -- Return/RConn1
  Flow after valve sensor/RConn2 -- Constant Volume Hydraulic Chamber/LConn1 -- From Valve/RConn1 -- Pressure after valve sensor/LConn1
  4-Way Directional Valve/RConn3 -- Hydraulic Reference3/LConn1
  From HPU/RConn1 -- Hydraulic Pressure Sensor2/LConn1 -- Flow through valve sensor/LConn1
  Constant Volume Hydraulic Chamber3/LConn1 -- 4-Way Directional Valve/LConn2 -- Hydraulic Flow Rate Sensor3/RConn2
  Flow after valve sensor/LConn1 -- 4-Way Directional Valve/LConn1 -- Hydraulic Pressure Sensor2/RConn1
  PS-Simulink Converter11/LConn1 -- Hydraulic Pressure Sensor2/RConn2
  4-Way Directional Valve/RConn1 -- Simulink-PS Converter4/RConn1
  Pressure after valve sensor/RConn1 -- Hydraulic Reference4/LConn1
  4-Way Directional Valve/RConn2 -- Flow through valve sensor/RConn2
  Pressure after valve sensor/RConn2 -- PS-Simulink Converter7/LConn1
  Flow after valve sensor/RConn1 -- PS-Simulink Converter6/LConn1
  Flow through valve sensor/RConn1 -- PS-Simulink Converter12/LConn1
  PS-Simulink Converter8/LConn1 -- Hydraulic Flow Rate Sensor3/RConn1
  Hydraulic Reference6/LConn1 -- Hydraulic Pressure Sensor3/RConn1
  PS-Simulink Converter16/LConn1 -- Hydraulic Pressure Sensor3/RConn2

== matlab function heaveCompMichael_v07/Control System/MATLAB Function4 ==
  data: t input; zp_ref output; zp_dot_ref output
function [zp_ref, zp_dot_ref]  = z_height(t)

z_w = 0.8; % m
T_w = 10; % s

zp_ref = z_w * sin((2*pi*t)/T_w);
zp_dot_ref = (2*z_w*pi*cos((2*pi*t)/T_w))/T_w;

== matlab function heaveCompMichael_v07/Control Signal/Variable pressure function ==
  data: u input; s output
function s = vp(u)

if(u > 0)
    s = 260e5;
else
    s = 120e5;
end

== matlab function heaveCompMichael_v07/Motor Brake/Brake valve control ==
  data: pressure1 input; u output; pressure2 input
function u = fcn(pressure1,pressure2)

p_cr = 20; % bar
dp_fo = 10; % bar, delta p_fully_open

u = (pressure1 - pressure2 - p_cr)/dp_fo;

== matlab function heaveCompMichael_v07/Motor/MATLAB Function7 ==
  data: t input; omega_m input; Mm output
function Mm = motor_moment(t, omega_m)

n_sh = 3; % shieves
i_g = 46; % gearbox ratio
m_pl = 9000; % kg
d_D = 0.45; % m
mu_eq = 0.15; % -
omega_0 = 5; % rad/s
g = 9.81; % m/(s^2)

if(t < 10^-3)
    omega_m = 0;
end

Mm = (m_pl*g*d_D)/(2*n_sh*2*i_g) * (1 + mu_eq * tanh(omega_m/omega_0));

== matlab function heaveCompMichael_v07/Control System/MATLAB Function8 ==
  data: zp_dot input; u output; n output; Q output
function [u, n, Q] = ff(zp_dot)

dd = 0.45;
rho = 875; % kg/m^3

Dm = 28.1*10^-6; % m^3/rev
n = (zp_dot/(dd/2)) * 46  * 6 / (2*pi); % rev/s

Q = (Dm*n);

Cd = 0.7;
Admax = (5.324e-5)*2; % m^2

u = (Q/(Cd*Admax * sqrt(2/rho*35e5))); % dp = p_mo = pressure metering orifice

% m/s
